simulink model "semi_GSTA"  (R2018b)
settings: Solver=FixedStepAuto  StartTime=0.0  StopTime=100  FixedStep=0.01  RelTol=1e-3
InitFcn:
  | parameters_semi_const_noise
model workspace: external: MAT-File (data not in the file)
undefined symbols (not defined in the file or in its folder): eta0, ev_sampling_time, fig_st, h_ATD, h_ATD_sds, Mn, st_controller, T0, v0, x1, x2, x3, x4, x5, x6
libraries: sdolib x6, simulink x1
(part 1 of 6)
settings Model: Creator=DING  LastModifiedBy=DNN
settings SolverCC: ZeroCrossAlgorithm=Adaptive
settings OptimizationCC: DefaultParameterBehavior=Inlined  EnhancedBackFolding=on  PassReuseOutputArgsAs=Individual arguments  MaxStackSize=64  OptimizeBlockOrder=speed  DifferentSizesBufferReuse=on  OptimizationCustomize=off
settings DebuggingCC: IgnoredZcDiagnostic=none  ParameterTunabilityLossMsg=error
settings HardwareCC: ProdBitPerPointer=32  ProdBitPerSizeT=32  ProdBitPerPtrDiffT=32  ProdLargestAtomicInteger=Long  ProdLargestAtomicFloat=Double  ProdWordSize=32  ProdHWDeviceType=ARM Compatible->ARM 11
settings SFSimCC: MATLABDynamicMemAlloc=off
settings RTWCC: SystemTargetFile=ert.tlc  TemplateMakefile=ert_default_tmf  GenerateReport=on  Toolchain=Catkin  IncludeHyperlinkInReport=on  LaunchReport=on  GenerateTraceInfo=on  GenerateTraceReport=on  GenerateTraceReportSl=on  GenerateTraceReportSf=on  GenerateTraceReportEml=on
settings CodeAppCC: ForceParamTrailComments=on  IgnoreCustomStorageClasses=off  OperatorAnnotations=on  SimulinkDataObjDesc=on  SFDataObjDesc=on  InsertBlockDesc=on
settings ERTTargetCC: ERTCustomFileTemplate=example_file_process.tlc

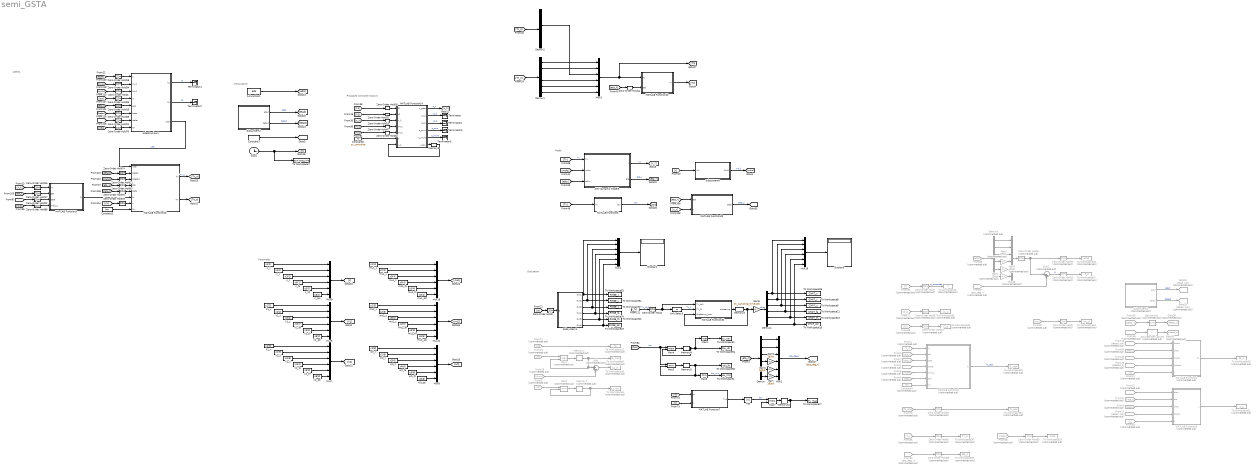
== system semi_GSTA ==
  note: Model
  note: Initialization
  note: Evaluation
  note: Proposed controller explicit
  note: Parameter
  note: AGSTA
  ARV Dynamic Model3 : Subsystem  VariantControl=Model_M
  Abs : Abs
  Adaptive law1 : Subsystem
  Add : Sum  Commented=on  Inputs=|+-
  Clock : Clock
  Constant1 : Constant  Value=[0 0 0 0 0 0]'
  Constant2 : Constant  Value=Mn  SampleTime=st_controller
  Constant4 : Constant  Commented=on  Value=Mn
  Constant8 : Constant  Value=st_controller  SampleTime=st_controller
  Demux{,1..2,4} (4 alike) : Demux  Outputs=6
  Demux5 : Demux  Commented=on  Outputs=6
  Derivative2 : Derivative  Commented=on
  Discrete Derivative1 : simulink/Discrete/Discrete Derivative  Commented=on  gainval=1.0  ICPrevScaledInput=0.0  OutMin=[]  OutMax=[]  OutDataType=fixdt(1, 16)  OutScaling=2^-10  DoSatur=off
  Display2 : Display
  Display6 : Display
  From11 : From  Commented=on  GotoTag=k0
  From12 : From  Commented=on  GotoTag=detad_sds
  From13 : From  Commented=on  GotoTag=etad_sds
  From15 : From  Commented=on  GotoTag=k1
  From17 : From  Commented=on  GotoTag=detad_sds
  From18 : From  Commented=on  GotoTag=c
  From19 : From  Commented=on  GotoTag=k1min
  From2 : From  Commented=on  GotoTag=ddeta_r
  From20 : From  Commented=on  GotoTag=ddetad_s
  From24 : From  Commented=on  GotoTag=c
  From{7,9,26,50} (4 alike) : From  Commented=on  GotoTag=deta_r
  From28 : From  Commented=on  GotoTag=mdis
  From3 : From  Commented=on  GotoTag=k1
  From4 : From  Commented=on  GotoTag=v_r
  From46 : From  Commented=on  GotoTag=detad_sds
  From47 : From  Commented=on  GotoTag=eta_r
  From48 : From  Commented=on  GotoTag=ddeta_r
  From5 : From  Commented=on  GotoTag=edis
  From54 : From  Commented=on  GotoTag=eta_deg_r
  From55 : From  Commented=on  GotoTag=Tv
  From6 : From  Commented=on  GotoTag=eta_r
  From60 : From  Commented=on  GotoTag=tou
  From61 : From  Commented=on  GotoTag=t
  From66 : From  Commented=on  GotoTag=etad
  From67 : From  Commented=on  GotoTag=eta_deg_r
  From69 : From  Commented=on  GotoTag=k2
  From70 : From  Commented=on  GotoTag=fx_eso
  From71 : From  Commented=on  GotoTag=k1
  From8 : From  Commented=on  GotoTag=mdis
  Gain : Gain  Gain=180/pi
  Gain1 : Gain  Gain=180/pi
  Gain2 : Gain  Gain=180/pi
  Gain4 : Gain  Commented=on  Gain=180/pi
  Gain5 : Gain  Commented=on  Gain=180/pi
  Gain6 : Gain  Gain=ev_sampling_time/100
  Gain7 : Gain  Commented=on  Gain=180/pi
  Goto28 : Goto  Commented=on  GotoTag=detad_sds
  Goto30 : Goto  Commented=on  GotoTag=etad_sds
  Goto35 : Goto  Commented=on  GotoTag=ddetad_s
  Goto38 : Goto  Commented=on  GotoTag=ddeta_r
  MATLAB Function10 : MATLAB Function  TreatAsAtomicUnit=on
  MATLAB Function14 : MATLAB Function  TreatAsAtomicUnit=on
  MATLAB Function15 : MATLAB Function  TreatAsAtomicUnit=on
  MATLAB Function2 : MATLAB Function  Commented=on  TreatAsAtomicUnit=on
  MATLAB Function20 : MATLAB Function  TreatAsAtomicUnit=on
  MATLAB Function3 : MATLAB Function  TreatAsAtomicUnit=on
  MATLAB Function31 : MATLAB Function  TreatAsAtomicUnit=on
  MATLAB Function4 : MATLAB Function  Commented=on  TreatAsAtomicUnit=on
  MATLAB Function5 : MATLAB Function  Commented=on  TreatAsAtomicUnit=on
  MATLAB Function6 : MATLAB Function  TreatAsAtomicUnit=on
  MATLAB Function7 : MATLAB Function  TreatAsAtomicUnit=on
  Max1 : MinMax  Commented=on  Function=max  Inputs=2
  Max2 : MinMax  Commented=on  Inputs=2
  Max3 : MinMax  Function=max
  Max4 : MinMax  Function=max  Inputs=2
  Max5 : MinMax  Inputs=2
  Max6 : MinMax
  Max7 : MinMax  Function=max  Inputs=2
  Memory10 : Memory  InheritSampleTime=on
  Memory2 : Memory  Commented=on
  Memory3 : Memory  InitialCondition=[0 0 0 0 0 0]  InheritSampleTime=on
  Memory4 : Memory  InheritSampleTime=on
  Memory5 : Memory  InheritSampleTime=on
  Memory7 : Memory  Commented=on  InitialCondition=100
  Memory8 : Memory  InitialCondition=[0 0 0 0 0 0]  InheritSampleTime=on
  Mux{1..3,6..9,18..19,21} (10 alike) : Mux  Inputs=6
  Mux25 : Mux  Commented=on  Inputs=6
  S-Function1 : S-Function  FunctionName=edis  SFunctionDeploymentMode=off  EnableBusSupport=off
  Subsystem1 : Subsystem
  Subsystem2 : Subsystem
  Subsystem3 : Subsystem  Commented=on
  Subsystem8 : Subsystem
  Sum2 : Sum  Commented=on  Inputs=|-+
  Terminator{,1..5} (6 alike) : Terminator
  To Workspace1 : ToWorkspace  VariableName=tou_min  SampleTime=-1
      settings: MaxDataPoints=1
  To Workspace10 : ToWorkspace  Commented=on  VariableName=k1_e  SampleTime=-1
      settings: MaxDataPoints=1
  To Workspace11 : ToWorkspace  VariableName=CHAT_fa  SampleTime=-1
      settings: MaxDataPoints=1
  To Workspace12 : ToWorkspace  Commented=on  VariableName=k0  SampleTime=-1
      settings: MaxDataPoints=1
  To Workspace13 : ToWorkspace  VariableName=CHAT_th  SampleTime=-1
      settings: MaxDataPoints=1
  To Workspace14 : ToWorkspace  Commented=on  VariableName=fx_eso  SampleTime=-1
  To Workspace15 : ToWorkspace  VariableName=CHAT_psi  SampleTime=-1
      settings: MaxDataPoints=1
  To Workspace16 : ToWorkspace  Commented=on  VariableName=fx_real  SampleTime=-1
  To Workspace17 : ToWorkspace  VariableName=Tv_max  SampleTime=-1
      settings: MaxDataPoints=1
  To Workspace18 : ToWorkspace  Commented=on  VariableName=mdis  SampleTime=-1
  To Workspace2 : ToWorkspace  VariableName=tou_max  SampleTime=-1
      settings: MaxDataPoints=1
  To Workspace21 : ToWorkspace  Commented=on  VariableName=s_p  SampleTime=-1
  To Workspace22 : ToWorkspace  VariableName=RMSE_th  SampleTime=-1
      settings: MaxDataPoints=1
  To Workspace23 : ToWorkspace  VariableName=RMSE_psi  SampleTime=-1
      settings: MaxDataPoints=1
  To Workspace24 : ToWorkspace  VariableName=RMSE_fa  SampleTime=-1
      settings: MaxDataPoints=1
  To Workspace25 : ToWorkspace  VariableName=CHAT_x  SampleTime=-1
      settings: MaxDataPoints=1
  To Workspace26 : ToWorkspace  Commented=on  VariableName=ds_p  SampleTime=-1
  To Workspace27 : ToWorkspace  VariableName=RMSE_z  SampleTime=-1
      settings: MaxDataPoints=1
  To Workspace29 : ToWorkspace  Commented=on  VariableName=etad  SampleTime=-1
  To Workspace3 : ToWorkspace  Commented=on  VariableName=k1_min  SampleTime=-1
      settings: MaxDataPoints=1
  To Workspace31 : ToWorkspace  Commented=on  VariableName=k2_p  SampleTime=-1
  To Workspace34 : ToWorkspace  Commented=on  VariableName=tou_p  SampleTime=-1
  To Workspace36 : ToWorkspace  Commented=on  VariableName=Tv_p  SampleTime=-1
  To Workspace37 : ToWorkspace  Commented=on  VariableName=e_p  SampleTime=-1
  To Workspace39 : ToWorkspace  Commented=on  VariableName=eta_p  SampleTime=-1
  To Workspace4 : ToWorkspace  Commented=on  VariableName=t  SampleTime=-1
  To Workspace53 : ToWorkspace  VariableName=RMSE_x  SampleTime=-1
      settings: MaxDataPoints=1
  To Workspace54 : ToWorkspace  VariableName=RMSE_y  SampleTime=-1
      settings: MaxDataPoints=1
  To Workspace55 : ToWorkspace  Commented=on  VariableName=k1_p  SampleTime=-1
  To Workspace6 : ToWorkspace  Commented=on  VariableName=k1_max  SampleTime=-1
      settings: MaxDataPoints=1
  To Workspace61 : ToWorkspace  VariableName=tou_ub  SampleTime=-1
      settings: MaxDataPoints=1
  To Workspace62 : ToWorkspace  VariableName=tou_lb  SampleTime=-1
      settings: MaxDataPoints=1
  To Workspace7 : ToWorkspace  VariableName=terminate_time  SampleTime=-1
      settings: MaxDataPoints=1
  To Workspace8 : ToWorkspace  VariableName=CHAT_y  SampleTime=-1
      settings: MaxDataPoints=1
  To Workspace9 : ToWorkspace  VariableName=CHAT_z  SampleTime=-1
      settings: MaxDataPoints=1
  Unit Delay3 : UnitDelay  SampleTime=ev_sampling_time
  Zero-Order Hold1 : ZeroOrderHold  SampleTime=ev_sampling_time
  Zero-Order Hold{5..10,12..13,55,57..58} (11 alike) : ZeroOrderHold  Commented=on  SampleTime=fig_st
  Zero-Order Hold{3,11,14..18,21..23,30..35,47,67..68,70,74..76} (23 alike) : ZeroOrderHold  SampleTime=st_controller
  Zero-Order Hold2 : ZeroOrderHold  SampleTime=ev_sampling_time
  c_fa : Constant  Value=x4(1)  VectorParams1D=off
  c_psi : Constant  Value=x6(1)
  c_th : Constant  Value=x5(1)
  c_x : Constant  Value=x1(1)
  c_y : Constant  Value=x2(1)  VectorParams1D=off
  c_z : Constant  Value=x3(1)
  k1_fa : Constant  Value=x4(2)
  k1_psi : Constant  Value=x6(2)
  k1_th : Constant  Value=x5(2)
  k1_x : Constant  Value=x1(2)
  k1_y : Constant  Value=x2(2)
  k1_z : Constant  Value=x3(2)
  k2_fa : Constant  Value=x4(3)
  k2_psi : Constant  Value=x6(3)
  k2_th : Constant  Value=x5(3)
  k2_x : Constant  Value=x1(3)
  k2_y : Constant  Value=x2(3)
  k2_z : Constant  Value=x3(3)
  mu1_fa : Constant  Value=x4(4)
  mu1_psi : Constant  Value=x6(4)
  mu1_th : Constant  Value=x5(4)
  mu1_x : Constant  Value=x1(4)  VectorParams1D=off
  mu1_y : Constant  Value=x2(4)
  mu1_z : Constant  Value=x3(4)
  mu2_fa : Constant  Value=x4(5)
  mu2_psi : Constant  Value=x6(5)
  mu2_th : Constant  Value=x5(5)
  mu2_x : Constant  Value=x1(5)
  mu2_y : Constant  Value=x2(5)
  mu2_z : Constant  Value=x3(5)
  w0_fa : Constant  Value=x4(6)
  w0_psi : Constant  Value=x6(6)
  w0_th : Constant  Value=x5(6)
  w0_x : Constant  Value=x1(6)
  w0_y : Constant  Value=x2(6)
  w0_z : Constant  Value=x3(6)
  wires:
  Constant1/1 -> [ddetad]
  ARV Dynamic Model3/2(eta) -> [eta_r]  "eta_r"
  Gain/1 -> Mux2/6
  Demux/6 -> Gain/1
  Gain1/1 -> Mux2/5
  Demux/5 -> Gain1/1
  Demux/4 -> Gain2/1
  Gain2/1 -> Mux2/4
  Demux/3 -> Mux2/3
  Demux/2 -> Mux2/2
  Demux/1 -> Mux2/1
  Max4/1 -> Memory4/1
  Memory5/1 -> To Workspace62/1, Max6/1, Max5/2
  [tou] -> Max4/1, Max5/1  "tou"
  Memory4/1 -> To Workspace61/1, Max3/1, Max4/2
  Max5/1 -> Memory5/1
  Mux2/1 -> [eta_deg_r]  "eta_deg_r"
  Demux4/3 -> To Workspace9/1, Mux19/3
  Mux19/1 -> Display6/1
  Demux4/1 -> To Workspace25/1, Mux19/1
  Demux4/4 -> To Workspace11/1, Mux19/4
  Demux4/5 -> To Workspace13/1, Mux19/5
  Demux4/6 -> To Workspace15/1, Mux19/6
  Demux4/2 -> To Workspace8/1, Mux19/2
  MATLAB Function6/1(tou) -> [tou]  "tou"
  Subsystem1/4(Out4) -> To Workspace24/1, Mux1/4
  MATLAB Function31/1(chattering) -> Memory3/1
  Gain6/1 -> Demux4/1  "chat"
  [Tv] -> Zero-Order Hold1/1  "Tv_k+1"
  Memory3/1 -> Gain6/1, MATLAB Function31/3(chattering_last)
  Unit Delay3/1 -> MATLAB Function31/2(Tv_k1)  "Tv_k"
  [e] -> Zero-Order Hold2/1
  Subsystem1/2(Out2) -> To Workspace54/1, Mux1/2
  Subsystem1/6(Out6) -> Mux1/6, To Workspace23/1
  Subsystem1/5(Out5) -> Mux1/5, To Workspace22/1
  Subsystem1/3(Out3) -> To Workspace27/1, Mux1/3
  Subsystem1/1(Out1) -> Mux1/1, To Workspace53/1
  Mux1/1 -> Display2/1
  [Tv] -> MATLAB Function6/1(Tv)
  Clock/1 -> To Workspace7/1, [t]
  Max6/1 -> To Workspace1/1  "tou_min"
  Max3/1 -> To Workspace2/1
  S-Function1/1 -> [edis]
  MATLAB Function20/1(deta) -> [deta_r]  "deta_r"
  [v_r] -> MATLAB Function20/2(v)
  [eta_r] -> MATLAB Function20/1(eta)
  ARV Dynamic Model3/1(v) -> [v_r]  "v_r"
  [eta_k] -> Demux/1
  Subsystem2/2(detad) -> [detad]  "detad"
  Subsystem2/1(etad) -> [etad]  "etad"
  Zero-Order Hold1/1 -> Unit Delay3/1, MATLAB Function31/1(Tv_kp1)
  Zero-Order Hold2/1 -> Subsystem1/1(e)
  [mdis] -> ARV Dynamic Model3/2(mdis)
  [Tv] -> ARV Dynamic Model3/1(Tv)  "Tv"
  [edis] -> ARV Dynamic Model3/3(edis)
  [t] -> Subsystem8/1(In1)
  Subsystem8/1(Out1) -> [mdis]  "mdis"
  Max1/1 -> Memory2/1
  Add/1 -> To Workspace10/1
  From15/1 -> Max1/1
  Memory2/1 -> To Workspace6/1, Max1/2, Add/1
  From19/1 -> Add/2
  From11/1 -> To Workspace12/1
  MATLAB Function14/1(u_gsta) -> [u_k]  "u_k"
  From3/1 -> Max2/1
  Max2/1 -> Memory7/1
  Memory7/1 -> To Workspace3/1, Max2/2
  From7/1 -> MATLAB Function2/3(deta)
  From28/1 -> Zero-Order Hold58/1
  Zero-Order Hold58/1 -> To Workspace18/1
  Zero-Order Hold57/1 -> To Workspace14/1
  Zero-Order Hold55/1 -> To Workspace39/1
  From61/1 -> Zero-Order Hold7/1
  Mux25/1 -> Zero-Order Hold5/1
  Zero-Order Hold6/1 -> To Workspace34/1
  From8/1 -> MATLAB Function2/5(mdis_c)
  Demux5/4 -> Gain7/1
  From6/1 -> MATLAB Function2/2(eta)
  Zero-Order Hold12/1 -> To Workspace29/1
  From17/1 -> MATLAB Function5/4(detad)
  Subsystem3/2(detad) -> Goto28/1  "detad"
  Demux5/6 -> Gain4/1
  Zero-Order Hold7/1 -> To Workspace4/1  "a_proposed"
  From46/1 -> Discrete Derivative1/1
  From13/1 -> MATLAB Function5/1(etad)
  From24/1 -> MATLAB Function4/5(c)
  MATLAB Function4/1(ds) -> To Workspace26/1
  Derivative2/1 -> Goto38/1
  MATLAB Function5/1(s) -> To Workspace21/1
  From18/1 -> MATLAB Function5/5(c)
  Demux5/5 -> Gain5/1
  From20/1 -> MATLAB Function4/4(ddetad)
  From47/1 -> MATLAB Function5/2(eta)
  From26/1 -> Derivative2/1
  Zero-Order Hold9/1 -> To Workspace55/1
  Zero-Order Hold8/1 -> To Workspace36/1
  From70/1 -> Zero-Order Hold57/1
  From12/1 -> MATLAB Function4/1(detad)
  Zero-Order Hold13/1 -> To Workspace37/1
  From71/1 -> Zero-Order Hold9/1
  From2/1 -> MATLAB Function2/4(ddeta)
  Demux5/1 -> Mux25/1
  Zero-Order Hold10/1 -> To Workspace31/1
  Subsystem3/1(etad) -> Goto30/1  "etad"
  Discrete Derivative1/1 -> Goto35/1
  From54/1 -> Zero-Order Hold55/1
  From50/1 -> MATLAB Function4/2(deta)
  From48/1 -> MATLAB Function4/3(ddeta)
  From69/1 -> Zero-Order Hold10/1
  From55/1 -> Zero-Order Hold8/1
  From9/1 -> MATLAB Function5/3(deta)
  Demux5/2 -> Mux25/2
  Constant4/1 -> MATLAB Function2/7(Mn)
  Zero-Order Hold5/1 -> Zero-Order Hold12/1, Sum2/1
  Sum2/1 -> Zero-Order Hold13/1  "e"
  From4/1 -> MATLAB Function2/1(vx)
  From66/1 -> Demux5/1
  From67/1 -> Sum2/2
  From5/1 -> MATLAB Function2/6(edis)
  Gain4/1 -> Mux25/6
  MATLAB Function2/1(fx) -> To Workspace16/1  "fx_real"
  From60/1 -> Zero-Order Hold6/1
  Demux5/3 -> Mux25/3
  Gain7/1 -> Mux25/4
  Gain5/1 -> Mux25/5
  [mu2] -> Zero-Order Hold32/1
  Mux18/1 -> [mu1]
  c_th/1 -> Mux9/5
  k2_x/1 -> Mux7/1
  mu1_th/1 -> Mux18/5
  c_z/1 -> Mux9/3
  [k1] -> Zero-Order Hold30/1
  w0_y/1 -> Mux8/2
  Mux7/1 -> [k2]
  mu1_z/1 -> Mux18/3
  w0_fa/1 -> Mux8/4
  k2_fa/1 -> Mux7/4
  MATLAB Function14/6(v_kp1) -> Memory8/1
  Zero-Order Hold30/1 -> MATLAB Function14/1(k1)
  k2_y/1 -> Mux7/2
  w0_x/1 -> Mux8/1
  mu1_fa/1 -> Mux18/4
  w0_th/1 -> Mux8/5
  mu1_x/1 -> Mux18/1
  [mu1] -> Zero-Order Hold47/1
  mu2_psi/1 -> Mux21/6
  k1_th/1 -> Mux6/5
  Mux21/1 -> [mu2]
  Mux6/1 -> [k1]
  mu1_y/1 -> Mux18/2
  mu1_psi/1 -> Mux18/6
  mu2_fa/1 -> Mux21/4
  k1_psi/1 -> Mux6/6
  c_y/1 -> Mux9/2
  k2_psi/1 -> Mux7/6
  c_x/1 -> Mux9/1
  mu2_z/1 -> Mux21/3
  mu2_th/1 -> Mux21/5
  k1_fa/1 -> Mux6/4
  k1_y/1 -> Mux6/2
  k2_th/1 -> Mux7/5
  Constant8/1 -> MATLAB Function14/6(h)
  Zero-Order Hold47/1 -> MATLAB Function14/4(mu1)
  mu2_y/1 -> Mux21/2
  k2_z/1 -> Mux7/3
  c_fa/1 -> Mux9/4
  k1_x/1 -> Mux6/1
  k1_z/1 -> Mux6/3
  mu2_x/1 -> Mux21/1
  Zero-Order Hold31/1 -> MATLAB Function14/2(k2)
  c_psi/1 -> Mux9/6
  Memory8/1 -> MATLAB Function14/7(v_k)
  Zero-Order Hold32/1 -> MATLAB Function14/5(mu2)
  w0_z/1 -> Mux8/3
  [k2] -> Zero-Order Hold31/1
  Mux9/1 -> [c]
  Mux8/1 -> [w0]
  w0_psi/1 -> Mux8/6
  [Tn_o] -> Demux1/1
  [Tn_p] -> Demux2/1
  Demux1/6 -> Mux3/6
  Mux3/1 -> [Tn], MATLAB Function10/1(Tn)
  [eta_k] -> Zero-Order Hold14/1
  MATLAB Function10/1(Tv) -> [Tv]
  Demux1/5 -> Mux3/5
  Demux1/2 -> Mux3/2
  Demux1/4 -> Mux3/4
  Zero-Order Hold14/1 -> MATLAB Function10/2(eta)
  Demux1/1 -> Mux3/1
  MATLAB Function14/2(u1_k) -> Terminator/1  "u1_k"
  MATLAB Function14/3(u2_k) -> Terminator1/1  "u2_k"
  MATLAB Function14/4(q_sum) -> Terminator3/1  "q_sum"
  MATLAB Function14/5(q_multi) -> Terminator5/1  "q_multi"
  [betax] -> Zero-Order Hold35/1
  [mu2x] -> Zero-Order Hold3/1
  [v_k] -> Zero-Order Hold16/1
  [mdis] -> Zero-Order Hold68/1
  Zero-Order Hold70/1 -> Adaptive law1/8(k0)
  Zero-Order Hold21/1 -> MATLAB Function15/3(ddetad)
  [wx] -> Zero-Order Hold33/1
  [cx] -> Zero-Order Hold76/1
  MATLAB Function3/1(fx) -> MATLAB Function15/6(fx)
  Adaptive law1/1(k1) -> Terminator4/1  "k1"
  [eta_k] -> Zero-Order Hold17/1
  Zero-Order Hold35/1 -> Adaptive law1/6(beta)
  Zero-Order Hold33/1 -> Adaptive law1/4(w)
  Zero-Order Hold74/1 -> MATLAB Function15/2(detad)
  [etad] -> Zero-Order Hold18/1
  [epsx] -> Zero-Order Hold15/1
  MATLAB Function15/1(Tv) -> [Tv_o]  "Tv_c"
  [deta_k] -> Zero-Order Hold22/1
  Zero-Order Hold22/1 -> MATLAB Function3/3(deta)
  Zero-Order Hold15/1 -> Adaptive law1/5(eps)
  Zero-Order Hold76/1 -> MATLAB Function15/7(c)
  Zero-Order Hold67/1 -> MATLAB Function15/4(eta)
  [detad] -> Zero-Order Hold74/1
  Adaptive law1/3(usta) -> MATLAB Function15/1(usta)  "usta"
  Zero-Order Hold3/1 -> Adaptive law1/3(mu2)
  [k0x] -> Zero-Order Hold70/1
  [ddetad] -> Zero-Order Hold21/1
  [deltax] -> Zero-Order Hold11/1
  Zero-Order Hold11/1 -> Adaptive law1/7(delta)
  [mu1x] -> Zero-Order Hold34/1
  Zero-Order Hold16/1 -> MATLAB Function3/1(vx)
  MATLAB Function15/2(Tn) -> [Tn_o]
  Adaptive law1/2(k2) -> Terminator2/1  "k2"
  Constant2/1 -> MATLAB Function15/8(Mn)
  Zero-Order Hold17/1 -> MATLAB Function3/2(eta)
  Zero-Order Hold75/1 -> MATLAB Function15/5(deta)
  [eta_k] -> Zero-Order Hold67/1
  Zero-Order Hold68/1 -> MATLAB Function3/4(mdis_c)
  Zero-Order Hold34/1 -> Adaptive law1/2(mu1)
  [deta_k] -> Zero-Order Hold75/1
  Demux2/3 -> Mux3/3
  MATLAB Function7/1(Tv0) -> Abs/1
  Max7/1 -> Memory10/1
  Abs/1 -> Max7/1  "tou"
  [t] -> MATLAB Function7/2(t)
  [Tv] -> MATLAB Function7/1(Tv)
  Memory10/1 -> To Workspace17/1, Max7/2
  Zero-Order Hold23/1 -> MATLAB Function14/3(x_k)
  [x_k] -> Zero-Order Hold23/1
  Zero-Order Hold18/1 -> Adaptive law1/1(s)

== system semi_GSTA/ARV Dynamic Model3 ==
  Tv : Inport
  mdis : Inport  Port=2
  edis : Inport  Port=3
  Constant : Constant  Commented=on  Value=0
  Demux : Demux  Outputs=6
  Integrator : Integrator  InitialCondition=v0
  Integrator1 : Integrator  InitialCondition=eta0
  MATLAB Function : MATLAB Function  TreatAsAtomicUnit=on
  Mux : Mux  Inputs=6
  v : Outport
  eta : Outport  Port=2
  wires:
  Integrator1/1 -> eta/1, MATLAB Function/5(eta)
  MATLAB Function/2(deta) -> Integrator1/1
  MATLAB Function/1(dv) -> Integrator/1
  edis/1 -> MATLAB Function/3(edis)
  mdis/1 -> MATLAB Function/2(mdis)
  Integrator/1 -> MATLAB Function/4(vx), v/1
  Tv/1 -> Demux/1
  Demux/3 -> Mux/3
  Demux/4 -> Mux/4
  Demux/5 -> Mux/5
  Mux/1 -> MATLAB Function/1(Tv)
  Demux/6 -> Mux/6
  Demux/2 -> Mux/2
  Demux/1 -> Mux/1

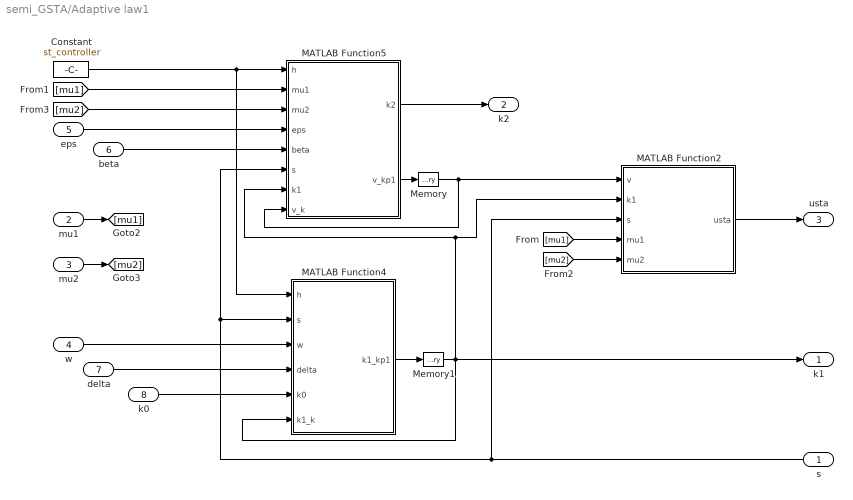
== system semi_GSTA/Adaptive law1 ==
  s : Inport
  mu1 : Inport  Port=2
  mu2 : Inport  Port=3
  w : Inport  Port=4
  eps : Inport  Port=5
  beta : Inport  Port=6
  delta : Inport  Port=7
  k0 : Inport  Port=8
  Constant : Constant  Value=st_controller  SampleTime=st_controller
  MATLAB Function2 : MATLAB Function  TreatAsAtomicUnit=on
  MATLAB Function4 : MATLAB Function  TreatAsAtomicUnit=on
  MATLAB Function5 : MATLAB Function  TreatAsAtomicUnit=on
  Memory : Memory  InitialCondition=[0 0 0 0 0 0]  InheritSampleTime=on
  Memory1 : Memory  InitialCondition=[0 0 0 0 0 0]  InheritSampleTime=on
  k1 : Outport
  k2 : Outport  Port=2
  usta : Outport  Port=3
  wires:
  Memory1/1 -> MATLAB Function2/2(k1), MATLAB Function5/7(k1), k1/1, MATLAB Function4/6(k1_k)
  [mu1] -> MATLAB Function5/2(mu1)
  eps/1 -> MATLAB Function5/4(eps)
  beta/1 -> MATLAB Function5/5(beta)
  [mu1] -> MATLAB Function2/4(mu1)
  w/1 -> MATLAB Function4/3(w)
  MATLAB Function5/1(k2) -> k2/1
  MATLAB Function4/1(k1_kp1) -> Memory1/1
  Memory/1 -> MATLAB Function2/1(v), MATLAB Function5/8(v_k)
  MATLAB Function5/2(v_kp1) -> Memory/1
  MATLAB Function2/1(usta) -> usta/1
  s/1 -> MATLAB Function2/3(s), MATLAB Function5/6(s), MATLAB Function4/2(s)
  Constant/1 -> MATLAB Function5/1(h), MATLAB Function4/1(h)
  [mu2] -> MATLAB Function2/5(mu2)
  [mu2] -> MATLAB Function5/3(mu2)
  mu1/1 -> [mu1]
  mu2/1 -> [mu2]
  delta/1 -> MATLAB Function4/4(delta)
  k0/1 -> MATLAB Function4/5(k0)

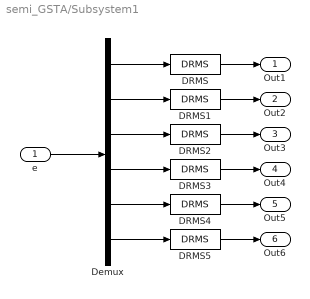
== system semi_GSTA/Subsystem1 ==
  e : Inport
  DRMS{,1..5} (6 alike) : sdolib/RMS Blocks/DRMS  Ts=ev_sampling_time
      settings: SourceProductBaseCode=SO
  Demux : Demux  Outputs=6
  Out1 : Outport
  Out2 : Outport  Port=2
  Out3 : Outport  Port=3
  Out4 : Outport  Port=4
  Out5 : Outport  Port=5
  Out6 : Outport  Port=6
  wires:
  e/1 -> Demux/1
  Demux/5 -> DRMS4/1
  Demux/3 -> DRMS2/1
  Demux/2 -> DRMS1/1
  Demux/4 -> DRMS3/1
  Demux/6 -> DRMS5/1
  Demux/1 -> DRMS/1
  DRMS/1 -> Out1/1
  DRMS1/1 -> Out2/1
  DRMS2/1 -> Out3/1
  DRMS3/1 -> Out4/1
  DRMS4/1 -> Out5/1
  DRMS5/1 -> Out6/1

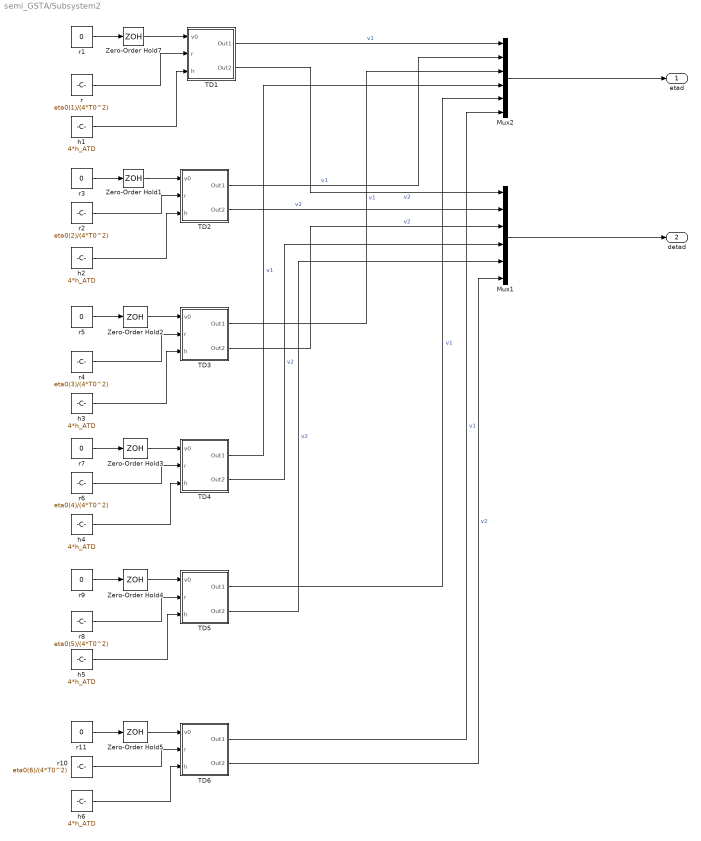
== system semi_GSTA/Subsystem2 ==
  Mux1 : Mux  Inputs=6
  Mux2 : Mux  Inputs=6
  TD1 : Subsystem
  TD2 : Subsystem
  TD3 : Subsystem
  TD4 : Subsystem
  TD5 : Subsystem
  TD6 : Subsystem
  Zero-Order Hold{1..5,7} (6 alike) : ZeroOrderHold  SampleTime=h_ATD
  h{1..6} (6 alike) : Constant  Value=4*h_ATD  SampleTime=h_ATD
  r : Constant  Value=eta0(1)/(4*T0^2)  SampleTime=h_ATD
  r{1,3,5,7,9,11} (6 alike) : Constant  Value=0  SampleTime=h_ATD
  r10 : Constant  Value=eta0(6)/(4*T0^2)  SampleTime=h_ATD
  r2 : Constant  Value=eta0(2)/(4*T0^2)  SampleTime=h_ATD
  r4 : Constant  Value=eta0(3)/(4*T0^2)  SampleTime=h_ATD
  r6 : Constant  Value=eta0(4)/(4*T0^2)  SampleTime=h_ATD
  r8 : Constant  Value=eta0(5)/(4*T0^2)  SampleTime=h_ATD
  etad : Outport
  detad : Outport  Port=2
  wires:
  r4/1 -> TD3/2(r)
  TD5/1(Out1) -> Mux2/5  "v1"
  TD6/1(Out1) -> Mux2/6  "v1"
  r8/1 -> TD5/2(r)
  TD2/1(Out1) -> Mux2/2  "v1"
  Zero-Order Hold3/1 -> TD4/1(v0)
  TD6/2(Out2) -> Mux1/6  "v2"
  r6/1 -> TD4/2(r)
  TD4/1(Out1) -> Mux2/4  "v1"
  TD1/1(Out1) -> Mux2/1  "v1"
  Zero-Order Hold1/1 -> TD2/1(v0)
  Zero-Order Hold4/1 -> TD5/1(v0)
  TD4/2(Out2) -> Mux1/4  "v2"
  Zero-Order Hold2/1 -> TD3/1(v0)
  Mux2/1 -> etad/1
  r10/1 -> TD6/2(r)
  TD2/2(Out2) -> Mux1/2  "v2"
  r7/1 -> Zero-Order Hold3/1
  h1/1 -> TD1/3(h)
  r11/1 -> Zero-Order Hold5/1
  Zero-Order Hold5/1 -> TD6/1(v0)
  r/1 -> TD1/2(r)
  r9/1 -> Zero-Order Hold4/1
  r3/1 -> Zero-Order Hold1/1
  TD1/2(Out2) -> Mux1/1  "v2"
  r2/1 -> TD2/2(r)
  Zero-Order Hold7/1 -> TD1/1(v0)
  r1/1 -> Zero-Order Hold7/1
  Mux1/1 -> detad/1
  TD5/2(Out2) -> Mux1/5  "v2"
  h2/1 -> TD2/3(h)
  h3/1 -> TD3/3(h)
  h4/1 -> TD4/3(h)
  h5/1 -> TD5/3(h)
  h6/1 -> TD6/3(h)
  r5/1 -> Zero-Order Hold2/1
  TD3/2(Out2) -> Mux1/3  "v2"
  TD3/1(Out1) -> Mux2/3  "v1"

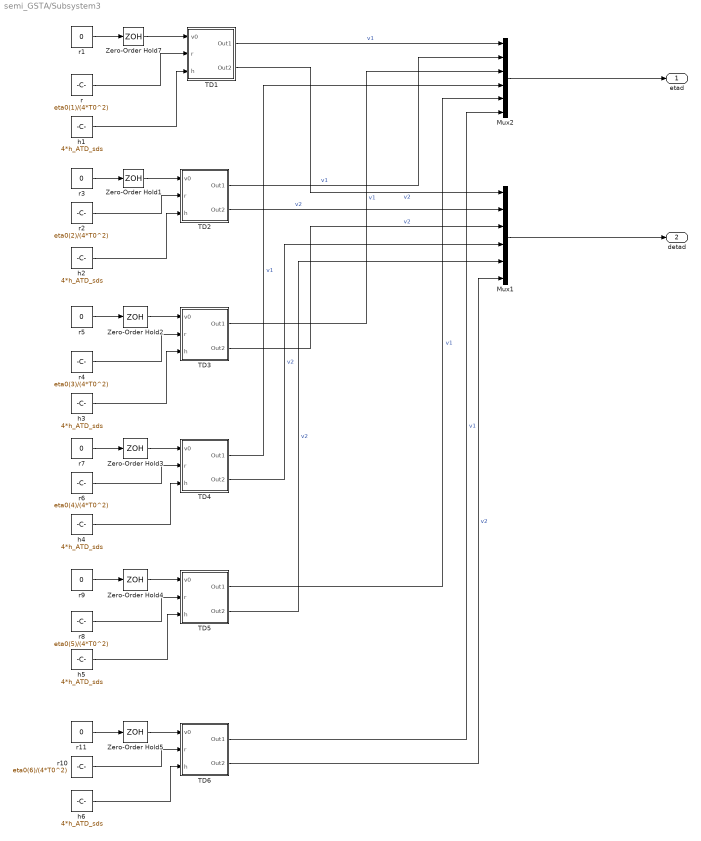
== system semi_GSTA/Subsystem3 ==
  Mux1 : Mux  Inputs=6
  Mux2 : Mux  Inputs=6
  TD1 : Subsystem
  TD2 : Subsystem
  TD3 : Subsystem
  TD4 : Subsystem
  TD5 : Subsystem
  TD6 : Subsystem
  Zero-Order Hold{1..5,7} (6 alike) : ZeroOrderHold  SampleTime=h_ATD_sds
  h{1..6} (6 alike) : Constant  Value=4*h_ATD_sds  SampleTime=h_ATD_sds
  r : Constant  Value=eta0(1)/(4*T0^2)  SampleTime=h_ATD_sds
  r{1,3,5,7,9,11} (6 alike) : Constant  Value=0  SampleTime=h_ATD_sds
  r10 : Constant  Value=eta0(6)/(4*T0^2)  SampleTime=h_ATD_sds
  r2 : Constant  Value=eta0(2)/(4*T0^2)  SampleTime=h_ATD_sds
  r4 : Constant  Value=eta0(3)/(4*T0^2)  SampleTime=h_ATD_sds
  r6 : Constant  Value=eta0(4)/(4*T0^2)  SampleTime=h_ATD_sds
  r8 : Constant  Value=eta0(5)/(4*T0^2)  SampleTime=h_ATD_sds
  etad : Outport
  detad : Outport  Port=2
  wires:
  TD3/1(Out1) -> Mux2/3  "v1"
  TD3/2(Out2) -> Mux1/3  "v2"
  r5/1 -> Zero-Order Hold2/1
  h6/1 -> TD6/3(h)
  h5/1 -> TD5/3(h)
  h4/1 -> TD4/3(h)
  h3/1 -> TD3/3(h)
  h2/1 -> TD2/3(h)
  TD5/2(Out2) -> Mux1/5  "v2"
  Mux1/1 -> detad/1
  r1/1 -> Zero-Order Hold7/1
  Zero-Order Hold7/1 -> TD1/1(v0)
  r2/1 -> TD2/2(r)
  TD1/2(Out2) -> Mux1/1  "v2"
  r3/1 -> Zero-Order Hold1/1
  r9/1 -> Zero-Order Hold4/1
  r/1 -> TD1/2(r)
  Zero-Order Hold5/1 -> TD6/1(v0)
  r11/1 -> Zero-Order Hold5/1
  h1/1 -> TD1/3(h)
  r7/1 -> Zero-Order Hold3/1
  TD2/2(Out2) -> Mux1/2  "v2"
  r10/1 -> TD6/2(r)
  Mux2/1 -> etad/1
  Zero-Order Hold2/1 -> TD3/1(v0)
  TD4/2(Out2) -> Mux1/4  "v2"
  Zero-Order Hold4/1 -> TD5/1(v0)
  Zero-Order Hold1/1 -> TD2/1(v0)
  TD1/1(Out1) -> Mux2/1  "v1"
  TD4/1(Out1) -> Mux2/4  "v1"
  r6/1 -> TD4/2(r)
  TD6/2(Out2) -> Mux1/6  "v2"
  Zero-Order Hold3/1 -> TD4/1(v0)
  TD2/1(Out1) -> Mux2/2  "v1"
  r8/1 -> TD5/2(r)
  TD6/1(Out1) -> Mux2/6  "v1"
  TD5/1(Out1) -> Mux2/5  "v1"
  r4/1 -> TD3/2(r)
